simulink model "complet_loesing"  (R2021b)
settings: Solver=FixedStepAuto  StartTime=0.0  StopTime=1000.0  FixedStep=0.002  MaxStep=0.02  MinStep=0.02  RelTol=1e-3  EnableMultiTasking=on
model workspace (MAT data in the model file):
  start_pos = 0
settings Model: Creator=shb  LastModifiedBy=klyx
settings SolverCC: AlgebraicLoopSolver=TrustRegion
settings DataIOCC: LimitDataPoints=on  SaveFormat=Array  ReturnWorkspaceOutputs=off
settings OptimizationCC: LifeSpan=inf
settings DebuggingCC: SFUnexpectedBacktrackingDiag=warning  SFNoUnconditionalDefaultTransitionDiag=warning  SFExecutionAtInitializationDiag=none  SFMachineParentedDataDiag=warning  ArithmeticOperatorsInVariantConditions=warning
settings HardwareCC: ProdBitPerPointer=32  ProdBitPerSizeT=32  ProdBitPerPtrDiffT=32  ProdLargestAtomicFloat=None  ProdIntDivRoundTo=Undefined  ProdEndianess=Unspecified  ProdWordSize=32  ProdHWDeviceType=32-bit Generic
settings ModelReferenceCC: PropagateSignalLabelsOutOfModel=off
settings SFSimCC: SimUseLocalCustomCode=off  CustomCodeUndefinedFunction=UseInterfaceOnly
settings RTWCC: RTWUseLocalCustomCode=off
settings CodeAppCC: StateflowObjectComments=on
settings GRTTargetCC: TargetLangStandard=C89/C90 (ANSI)
settings ConfigComp: CovMetricSettings=dw  CovSaveCumulativeToWorkspaceVar=on  CovSaveSingleToWorkspaceVar=on  CovExternalEMLEnable=off

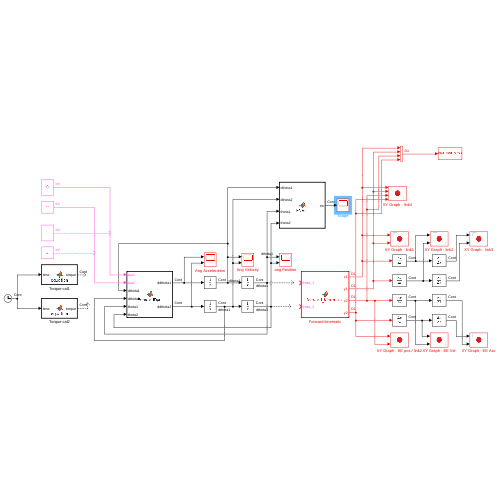
[thumbnail: Simulink's stored preview of the top-level diagram]
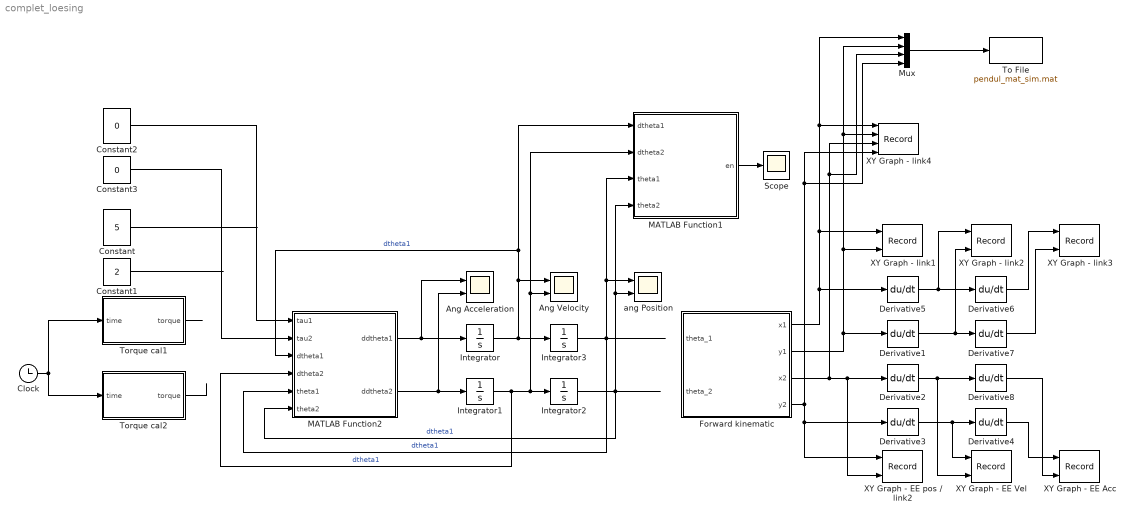
== system complet_loesing ==
  Ang Acceleration : Scope  NumInputPorts=2
  Ang Velocity : Scope  NumInputPorts=2
  Clock : Clock
  Constant : Constant  Value=5
  Constant1 : Constant  Value=2
  Constant2 : Constant  Value=0
  Constant3 : Constant  Value=0
  Derivative{1..8} (8 alike) : Derivative
  Forward kinematic : MATLAB Function  TreatAsAtomicUnit=on
  Integrator : Integrator
  Integrator1 : Integrator
  Integrator2 : Integrator
  Integrator3 : Integrator  InitialCondition=pi*6/4+0.7
  MATLAB Function1 : MATLAB Function  TreatAsAtomicUnit=on
  MATLAB Function2 : MATLAB Function  TreatAsAtomicUnit=on
  Mux : Mux
  Scope : Scope
  To File : ToFile  Filename=pendul_mat_sim.mat
      settings: Decimation=4
  Torque cal1 : MATLAB Function  TreatAsAtomicUnit=on
  Torque cal2 : MATLAB Function  TreatAsAtomicUnit=on
  XY Graph - EE Acc : Record  FileSettingsInternal="{\"entries\":[{\"content\":{\"excelSettings\":{\"content\":{},\"type\":\"Streamout.ExcelSettings\"}},\"type\":\"Streamout.FileSettingStorage\",\"uuid\":\"d6aca283-fdff-48c4-8fcc-4ce8f09bde04\"}],\"packageUris\":[\"http://schema.mathworks.com/mf0/streamout_blocks/R2020a\"],\"version\":\"1.0\"}"  Layout=[1 1]  SignalsInternal="{\"entries\":[{\"content\":{\"signals\":[{\"content\":{\"blockPath\":[\"complet_loesing/XY Graph - EE Acc\"],\"channel\":[],\"dimensions\":[1],\"domain\":\"complet_loesing/XY Graph - EE Acc\",\"lineColor\":\"#77ac30\",\"plots\":[1],\"port\":1,\"sid\":[\"\"],\"signalID\":100113,\"signalName\":\"Derivative4\"},\"type\":\"RecordBlkView.Signal\",\"uuid\":\"afbcaff0-f686-4179-a59e-e841b38025bd\"},{\"content\":{\"blockPath\":[\"complet_loesing/XY Graph - EE Acc\"],\"channel\":[],\"dimensions\":[1],\"domain\":\"complet_loesing/XY Graph - EE Acc\",\"lineColor\":\"#4dbeee\",\"plots\":[1],\"port\":2,\"sid\":[\"\"],\"signalID\":100117,\"signalName\":\"Derivative8\"},\"type\":\"RecordBlkView.Signal\",\"uuid\":\"9dac792e-41e9-49bb-a165-beab4b14f6cb\"}]},\"type\":\"RecordBlkView.InputSignals\",\"uuid\":\"44131724-f22f-4265-9c9f-93120ac999df\"}],\"packageUris\":[\"http://schema.mathworks.com/mf0/streamout_blocks/R2020a\"],\"version\":\"1.0\"}"  VisualizationBindings="{\"xyplotplugin\":{\"info\":[{\"series\":[{\"bindingParametersList\":[{\"parameter\":\"Y-Axis\",\"signalID\":100117,\"signalName\":\"Derivative8\"},{\"parameter\":\"X-Axis\",\"signalID\":100113,\"signalName\":\"Derivative4\"}],\"seriesID\":2515}],\"subplotID\":1}]}}"  CompatibilityTag=XY
  XY Graph - EE Vel : Record  FileSettingsInternal="{\"entries\":[{\"content\":{\"excelSettings\":{\"content\":{},\"type\":\"Streamout.ExcelSettings\"}},\"type\":\"Streamout.FileSettingStorage\",\"uuid\":\"c1cbff45-cac1-4d4b-9f4e-b6693e3c3237\"}],\"packageUris\":[\"http://schema.mathworks.com/mf0/streamout_blocks/R2020a\"],\"version\":\"1.0\"}"  Layout=[1 1]  SignalsInternal="{\"entries\":[{\"content\":{\"signals\":[{\"content\":{\"blockPath\":[\"complet_loesing/XY Graph - EE Vel\"],\"channel\":[],\"dimensions\":[1],\"domain\":\"complet_loesing/XY Graph - EE Vel\",\"lineColor\":\"#a2142f\",\"plots\":[1],\"port\":1,\"sid\":[\"\"],\"signalID\":100121,\"signalName\":\"Derivative3\"},\"type\":\"RecordBlkView.Signal\",\"uuid\":\"93be86fa-b32d-43c6-85ba-361e484ae1e0\"},{\"content\":{\"blockPath\":[\"complet_loesing/XY Graph - EE Vel\"],\"channel\":[],\"dimensions\":[1],\"domain\":\"complet_loesing/XY Graph - EE Vel\",\"lineColor\":\"#139fff\",\"plots\":[1],\"port\":2,\"sid\":[\"\"],\"signalID\":100125,\"signalName\":\"Derivative2\"},\"type\":\"RecordBlkView.Signal\",\"uuid\":\"ac2b6016-b468-4953-bc9b-5a3c7f3f7d47\"}]},\"type\":\"RecordBlkView.InputSignals\",\"uuid\":\"aaceb0ed-072a-49c4-a112-9adfbaa2f2ef\"}],\"packageUris\":[\"http://schema.mathworks.com/mf0/streamout_blocks/R2020a\"],\"version\":\"1.0\"}"  VisualizationBindings="{\"xyplotplugin\":{\"info\":[{\"series\":[{\"bindingParametersList\":[{\"parameter\":\"Y-Axis\",\"signalID\":100125,\"signalName\":\"Derivative2\"},{\"parameter\":\"X-Axis\",\"signalID\":100121,\"signalName\":\"Derivative3\"}],\"seriesID\":64261}],\"subplotID\":1}]}}"  CompatibilityTag=XY
  XY Graph - EE pos / link2 : Record  FileSettingsInternal="{\"entries\":[{\"content\":{\"excelSettings\":{\"content\":{},\"type\":\"Streamout.ExcelSettings\"}},\"type\":\"Streamout.FileSettingStorage\",\"uuid\":\"bb01f4bd-601a-486b-9bf1-6dc1eb75826c\"}],\"packageUris\":[\"http://schema.mathworks.com/mf0/streamout_blocks/R2020a\"],\"version\":\"1.0\"}"  Layout=[1 1]  SignalsInternal="{\"entries\":[{\"content\":{\"signals\":[{\"content\":{\"blockPath\":[\"complet_loesing/XY Graph - EE pos // link2\"],\"channel\":[],\"dimensions\":[1],\"domain\":\"complet_loesing/XY Graph - EE pos // link2\",\"lineColor\":\"#ff6929\",\"plots\":[1],\"port\":1,\"sid\":[\"\"],\"signalID\":100129,\"signalName\":\"Forward kinematic:4\"},\"type\":\"RecordBlkView.Signal\",\"uuid\":\"b0dcdc60-c7e2-4821-a3e0-0a64c6fe77f1\"},{\"content\":{\"blockPath\":[\"complet_loesing/XY Graph - EE pos // link2\"],\"channel\":[],\"dimensions\":[1],\"domain\":\"complet_loesing/XY Graph - EE pos // link2\",\"lineColor\":\"#b746ff\",\"plots\":[1],\"port\":2,\"sid\":[\"\"],\"signalID\":100133,\"signalName\":\"Forward kinematic:3\"},\"type\":\"RecordBlkView.Signal\",\"uuid\":\"ebf17f91-4ec2-4a28-8e83-7fdde1d74585\"}]},\"type\":\"RecordBlkView.InputSignals\",\"uuid\":\"4c935a8f-429f-4dfa-b09f-879e66123d81\"}],\"packageUris\":[\"http://schema.mathworks.com/mf0/streamout_blocks/R2020a\"],\"version\":\"1.0\"}"  VisualizationBindings="{\"xyplotplugin\":{\"info\":[{\"series\":[{\"bindingParametersList\":[{\"parameter\":\"Y-Axis\",\"signalID\":100129,\"signalName\":\"Forward kinematic:4\"},{\"parameter\":\"X-Axis\",\"signalID\":100133,\"signalName\":\"Forward kinematic:3\"}],\"seriesID\":53260}],\"subplotID\":1}]}}"  CompatibilityTag=XY
  XY Graph - link1 : Record  FileSettingsInternal="{\"entries\":[{\"content\":{\"excelSettings\":{\"content\":{},\"type\":\"Streamout.ExcelSettings\"}},\"type\":\"Streamout.FileSettingStorage\",\"uuid\":\"fdac7daa-c8a3-4540-abb4-4f49f504efc3\"}],\"packageUris\":[\"http://schema.mathworks.com/mf0/streamout_blocks/R2020a\"],\"version\":\"1.0\"}"  Layout=[1 1]  SignalsInternal="{\"entries\":[{\"content\":{\"signals\":[{\"content\":{\"blockPath\":[\"complet_loesing/XY Graph - link1\"],\"channel\":[],\"dimensions\":[1],\"domain\":\"complet_loesing/XY Graph - link1\",\"lineColor\":\"#64d413\",\"plots\":[1],\"port\":1,\"sid\":[\"\"],\"signalID\":100137,\"signalName\":\"Forward kinematic:1\"},\"type\":\"RecordBlkView.Signal\",\"uuid\":\"8fab0f3d-3d5b-4d6b-8ac4-e270d178e799\"},{\"content\":{\"blockPath\":[\"complet_loesing/XY Graph - link1\"],\"channel\":[],\"dimensions\":[1],\"domain\":\"complet_loesing/XY Graph - link1\",\"lineColor\":\"#ff13a6\",\"plots\":[1],\"port\":2,\"sid\":[\"\"],\"signalID\":100141,\"signalName\":\"Forward kinematic:2\"},\"type\":\"RecordBlkView.Signal\",\"uuid\":\"d6e3aa42-bc67-491a-83cb-c8ee221d3fa1\"}]},\"type\":\"RecordBlkView.InputSignals\",\"uuid\":\"409af8a8-dd8e-4d71-bb1c-7ac8a9ec8ed8\"}],\"packageUris\":[\"http://schema.mathworks.com/mf0/streamout_blocks/R2020a\"],\"version\":\"1.0\"}"  VisualizationBindings="{\"xyplotplugin\":{\"info\":[{\"series\":[{\"bindingParametersList\":[{\"parameter\":\"Y-Axis\",\"signalID\":100141,\"signalName\":\"Forward kinematic:2\"},{\"parameter\":\"X-Axis\",\"signalID\":100137,\"signalName\":\"Forward kinematic:1\"}],\"seriesID\":2133}],\"subplotID\":1}]}}"  CompatibilityTag=XY
  XY Graph - link2 : Record  FileSettingsInternal="{\"entries\":[{\"content\":{\"excelSettings\":{\"content\":{},\"type\":\"Streamout.ExcelSettings\"}},\"type\":\"Streamout.FileSettingStorage\",\"uuid\":\"b236a057-b99d-41c6-a6e5-e83b1a5b8706\"}],\"packageUris\":[\"http://schema.mathworks.com/mf0/streamout_blocks/R2020a\"],\"version\":\"1.0\"}"  Layout=[1 1]  SignalsInternal="{\"entries\":[{\"content\":{\"signals\":[{\"content\":{\"blockPath\":[\"complet_loesing/XY Graph - link2\"],\"channel\":[],\"dimensions\":[1],\"domain\":\"complet_loesing/XY Graph - link2\",\"lineColor\":\"#64d413\",\"plots\":[1],\"port\":1,\"sid\":[\"\"],\"signalID\":100145,\"signalName\":\"Derivative5\"},\"type\":\"RecordBlkView.Signal\",\"uuid\":\"5b09d620-3109-4403-8167-03cf49e27985\"},{\"content\":{\"blockPath\":[\"complet_loesing/XY Graph - link2\"],\"channel\":[],\"dimensions\":[1],\"domain\":\"complet_loesing/XY Graph - link2\",\"lineColor\":\"#ff13a6\",\"plots\":[1],\"port\":2,\"sid\":[\"\"],\"signalID\":100149,\"signalName\":\"Derivative1\"},\"type\":\"RecordBlkView.Signal\",\"uuid\":\"8d21d701-1762-455d-8826-6f981b3b64f7\"}]},\"type\":\"RecordBlkView.InputSignals\",\"uuid\":\"aea57c56-e45f-46e7-a72c-03ae975a7b26\"}],\"packageUris\":[\"http://schema.mathworks.com/mf0/streamout_blocks/R2020a\"],\"version\":\"1.0\"}"  VisualizationBindings="{\"xyplotplugin\":{\"info\":[{\"series\":[{\"bindingParametersList\":[{\"parameter\":\"Y-Axis\",\"signalID\":100149,\"signalName\":\"Derivative1\"},{\"parameter\":\"X-Axis\",\"signalID\":100145,\"signalName\":\"Derivative5\"}],\"seriesID\":38942}],\"subplotID\":1}]}}"  CompatibilityTag=XY
  XY Graph - link3 : Record  FileSettingsInternal="{\"entries\":[{\"content\":{\"excelSettings\":{\"content\":{},\"type\":\"Streamout.ExcelSettings\"}},\"type\":\"Streamout.FileSettingStorage\",\"uuid\":\"cf77b2de-b438-4fb8-b814-05d167173ea0\"}],\"packageUris\":[\"http://schema.mathworks.com/mf0/streamout_blocks/R2020a\"],\"version\":\"1.0\"}"  Layout=[1 1]  SignalsInternal="{\"entries\":[{\"content\":{\"signals\":[{\"content\":{\"blockPath\":[\"complet_loesing/XY Graph - link3\"],\"channel\":[],\"dimensions\":[1],\"domain\":\"complet_loesing/XY Graph - link3\",\"lineColor\":\"#64d413\",\"plots\":[1],\"port\":1,\"sid\":[\"\"],\"signalID\":100153,\"signalName\":\"Derivative6\"},\"type\":\"RecordBlkView.Signal\",\"uuid\":\"2b66a1a0-ac9f-4455-b7e3-0ac80a6b8e90\"},{\"content\":{\"blockPath\":[\"complet_loesing/XY Graph - link3\"],\"channel\":[],\"dimensions\":[1],\"domain\":\"complet_loesing/XY Graph - link3\",\"lineColor\":\"#ff13a6\",\"plots\":[1],\"port\":2,\"sid\":[\"\"],\"signalID\":100157,\"signalName\":\"Derivative7\"},\"type\":\"RecordBlkView.Signal\",\"uuid\":\"0499e878-8dbd-4467-b495-b17744a1559b\"}]},\"type\":\"RecordBlkView.InputSignals\",\"uuid\":\"894e425a-12c6-4922-89de-6764b04aa296\"}],\"packageUris\":[\"http://schema.mathworks.com/mf0/streamout_blocks/R2020a\"],\"version\":\"1.0\"}"  VisualizationBindings="{\"xyplotplugin\":{\"info\":[{\"series\":[{\"bindingParametersList\":[{\"parameter\":\"Y-Axis\",\"signalID\":100157,\"signalName\":\"Derivative7\"},{\"parameter\":\"X-Axis\",\"signalID\":100153,\"signalName\":\"Derivative6\"}],\"seriesID\":1602}],\"subplotID\":1}]}}"  CompatibilityTag=XY
  XY Graph - link4 : Record  FileSettingsInternal="{\"entries\":[{\"content\":{\"excelSettings\":{\"content\":{},\"type\":\"Streamout.ExcelSettings\"}},\"type\":\"Streamout.FileSettingStorage\",\"uuid\":\"bdba9047-f3ad-43e2-a51a-1e47254a6cc4\"}],\"packageUris\":[\"http://schema.mathworks.com/mf0/streamout_blocks/R2020a\"],\"version\":\"1.0\"}"  Layout=[1 1]  SignalsInternal="{\"entries\":[{\"content\":{\"signals\":[{\"content\":{\"blockPath\":[\"complet_loesing/XY Graph - link4\"],\"channel\":[],\"dimensions\":[1],\"domain\":\"complet_loesing/XY Graph - link4\",\"lineColor\":\"#64d413\",\"plots\":[1],\"port\":1,\"sid\":[\"\"],\"signalID\":100161,\"signalName\":\"Forward kinematic:1\"},\"type\":\"RecordBlkView.Signal\",\"uuid\":\"8565c91b-6340-4e0f-8e60-cfd1f2052b5b\"},{\"content\":{\"blockPath\":[\"complet_loesing/XY Graph - link4\"],\"channel\":[],\"dimensions\":[1],\"domain\":\"complet_loesing/XY Graph - link4\",\"lineColor\":\"#ff13a6\",\"plots\":[1],\"port\":2,\"sid\":[\"\"],\"signalID\":100165,\"signalName\":\"Forward kinematic:2\"},\"type\":\"RecordBlkView.Signal\",\"uuid\":\"4216d971-aa50-41d7-be4d-17ef60a8742e\"},{\"content\":{\"blockPath\":[\"complet_loesing/XY Graph - link4\"],\"channel\":[],\"dimensions\":[1],\"domain\":\"complet_loesing/XY Graph - link4\",\"lineColor\":\"#ff6929\",\"plots\":[1],\"port\":3,\"sid\":[\"\"],\"signalID\":100169,\"signalName\":\"Forward kinematic:3\"},\"type\":\"RecordBlkView.Signal\",\"uuid\":\"7fea9a7c-f978-4b7a-9c5f-ad64dff34a17\"},{\"content\":{\"blockPath\":[\"complet_loesing/XY Graph - link4\"],\"channel\":[],\"dimensions\":[1],\"domain\":\"complet_loesing/XY Graph - link4\",\"lineColor\":\"#b746ff\",\"plots\":[1],\"port\":4,\"sid\":[\"\"],\"signalID\":100173,\"signalName\":\"Forward kinematic:4\"},\"type\":\"RecordBlkView.Signal\",\"uuid\":\"209b15a5-f09b-468f-877b-de2f1fdc3b04\"}]},\"type\":\"RecordBlkView.InputSignals\",\"uuid\":\"012b4deb-d0a5-471e-b189-85ebaab05d15\"}],\"packageUris\":[\"http://schema.mathworks.com/mf0/streamout_blocks/R2020a\"],\"version\":\"1.0\"}"  VisualizationBindings="{\"xyplotplugin\":{\"info\":[{\"series\":[{\"bindingParametersList\":[{\"parameter\":\"Y-Axis\",\"signalID\":100173,\"signalName\":\"Forward kinematic:4\"},{\"parameter\":\"X-Axis\",\"signalID\":100169,\"signalName\":\"Forward kinematic:3\"}],\"seriesID\":58674},{\"bindingParametersList\":[{\"parameter\":\"Y-Axis\",\"signalID\":100165,\"signalName\":\"Forward kinematic:2\"},{\"parameter\":\"X-Axis\",\"signalID\":100161,\"signalName\":\"Forward kinematic:1\"}],\"seriesID\":58351}],\"subplotID\":1}]}}"  CompatibilityTag=XY
  ang Position : Scope  NumInputPorts=2
  wires:
  MATLAB Function2/1(ddtheta1) -> Ang Acceleration/1, Integrator/1
  MATLAB Function2/2(ddtheta2) -> Ang Acceleration/2, Integrator1/1
  Integrator/1 -> MATLAB Function1/1(dtheta1), MATLAB Function2/3(dtheta1), Ang Velocity/1, Integrator3/1  "dtheta1"
  Integrator1/1 -> MATLAB Function1/2(dtheta2), Ang Velocity/2, Integrator2/1, MATLAB Function2/4(dtheta2)  "dtheta1"
  Integrator3/1 -> MATLAB Function1/3(theta1), ang Position/1, MATLAB Function2/5(theta1)  "dtheta1"
  Integrator2/1 -> MATLAB Function1/4(theta2), ang Position/2, MATLAB Function2/6(theta2)  "dtheta1"
  Constant1/1 -> ?
  Constant/1 -> ?
  Derivative8/1 -> XY Graph - EE Acc/2
  Derivative4/1 -> XY Graph - EE Acc/1
  Derivative2/1 -> XY Graph - EE Vel/2, Derivative8/1
  Derivative3/1 -> XY Graph - EE Vel/1, Derivative4/1
  Clock/1 -> Torque cal2/1(time), Torque cal1/1(time)
  Torque cal1/1(torque) -> ?
  Torque cal2/1(torque) -> ?
  Forward kinematic/1(x1) -> Derivative5/1, Mux/1, XY Graph - link4/1, XY Graph - link1/1
  Forward kinematic/2(y1) -> Derivative1/1, Mux/2, XY Graph - link4/2, XY Graph - link1/2
  Derivative1/1 -> XY Graph - link2/2, Derivative7/1
  Derivative5/1 -> XY Graph - link2/1, Derivative6/1
  Derivative7/1 -> XY Graph - link3/2
  Derivative6/1 -> XY Graph - link3/1
  Forward kinematic/4(y2) -> Mux/4, XY Graph - link4/4, XY Graph - EE pos / link2/1, Derivative3/1
  Constant2/1 -> MATLAB Function2/1(tau1)
  Constant3/1 -> MATLAB Function2/2(tau2)
  Forward kinematic/3(x2) -> Mux/3, XY Graph - link4/3, Derivative2/1, XY Graph - EE pos / link2/2
  Mux/1 -> To File/1
  MATLAB Function1/1(en) -> Scope/1

== matlab function complet_loesing/Torque cal1 ==
  data: time input; torque output
function torque = equation(time)

if time < 3
    torque = time*2;
elseif time < 6    
    torque= -2*time+12; 
else
    torque = 0;
end

== matlab function complet_loesing/Torque cal2 ==
  data: time input; torque output
function torque = equation(time)

if time < 3
    torque = time*1.166;
elseif time < 6    
    torque= -1.166*time+7; 
else
    torque = 0;
end

== matlab function complet_loesing/MATLAB Function2 ==
  data: tau1 input; ddtheta1 output; ddtheta2 output; tau2 input; dtheta1 input; dtheta2 input; theta1 input; theta2 input
function [ddtheta1, ddtheta2]= ForwardDyn(tau1, tau2, dtheta1, dtheta2, theta1, theta2)  

g = 9.81;
p = 7806;

l1 = 1;
lc1 = l1/2; %mas siger
l2 = 0.5;
lc2 = l2/2;
m1 = 0.05*0.05*l1*p; 
m2 = 0.05*0.05*l2*p;
I1 = m1*l1*l1/3;
I2 = m2*l2*l2/12;

H11 = m1*lc1*lc1+I1+I2+m2*(l1*l1+lc2*lc2+2*l1*lc2*cos(theta2));
H22 = m1*lc2*lc2+I2;
%H22 = m2*lc2*lc2+I2;
H12 = m2*(lc2*lc2+2*l1*lc2*cos(theta2))+I2;
h = m2*l1*lc2*sin(theta2);
G1 = m1*g*lc1*cos(theta1)+m2*g*(l1*cos(theta1)+lc2*cos(theta1+theta2));
G2 = m2*g*lc2*cos(theta1+theta2); 

% tau
tau = [tau1;tau2];
% H(theta)
M = [H11,H12;H12,H22];
%V ( theta dtheta)
V = [(-h*dtheta2*dtheta2-2*h*dtheta1*dtheta2);h*dtheta1*dtheta1];
% G( theta )
G = [G1;G2];
ddtheta = M\(tau-(V+G));
%ddtheta = inv(M)*(tau-(V+G));
%ddtheta = ddtheta;
ddtheta1 = ddtheta(1);
ddtheta2 = ddtheta(2);
%theta1 = (H11*ddtheta1 + H12*ddtheta2 - h*dtheta2*dtheta2 - 2*h*dtheta1*dtheta2 +G1)\u(1);
%theta1 = (H12*ddtheta1 + H22*ddtheta2 + h*dtheta2*dtheta2+G2)\u(2);

== matlab function complet_loesing/Forward kinematic ==
  data: theta_1 input; x1 output; y1 output; theta_2 input; x2 output; y2 output
function [x1, y1,x2,y2]=  forward_Kinematic(theta_1, theta_2)

l1 = 1;
l2 = 0.5;
x1 = l1*cos(theta_1);
y1 = l1*sin(theta_1);
x2 = l2*cos(theta_1+theta_2) +x1;
y2 = l2*sin(theta_1+theta_2)+ y1;

== matlab function complet_loesing/MATLAB Function1 ==
  data: en output; dtheta1 input; dtheta2 input; theta1 input; theta2 input
function en = ENAGI(dtheta1, dtheta2, theta1, theta2)  

g = 9.81;
p = 7806;

l1 = 1;
lc1 = l1/2; %mas siger
l2 = 0.5;
lc2 = l2/2;
m1 = 0.05*0.05*l1*p; 
m2 = 0.05*0.05*l2*p;
I1 = m1*l1*l1/3;
I2 = m2*l2*l2/12;

Vc2 = [-l1*dtheta1*sin(theta1)-lc2*(dtheta1+dtheta2)*sin(theta1+theta2);
    l1*dtheta1*cos(theta1)+lc2*(dtheta1+dtheta2)*cos(theta1+theta2)];
T1 = 0.5*dtheta1*dtheta1*(m1*lc1*lc1+I1);
V1 = m1*g*lc1*sin(theta1);
T2 = 0.5*I2*(dtheta1 + dtheta2)*(dtheta1 + dtheta2)+0.5*m2*dot(Vc2,Vc2);
V2 = m2*g*(l1*sin(theta1)+l2*sin(theta1+theta2));
%dot(Vc2,Vc2)
en = T1+- V1 + T2 + V2;
